simulink model "crc_8_general_manual"  (R2021b)
settings: Solver=FixedStepDiscrete  StartTime=0.0  StopTime=0.01  FixedStep=0.01  RelTol=1e-3
libraries: msbUtilities x9, commcrc2 x1
settings Model: Creator=jekyll  LastModifiedBy=jekyll
settings OptimizationCC: DefaultParameterBehavior=Inlined  EnhancedBackFolding=on  PassReuseOutputArgsAs=Individual arguments  OptimizeBlockOrder=speed  DifferentSizesBufferReuse=on  OptimizationCustomize=off  EfficientTunableParamExpr=on
settings DebuggingCC: ParameterTunabilityLossMsg=error
settings SFSimCC: MATLABDynamicMemAlloc=off
settings RTWCC: Description=Embedded Coder  SystemTargetFile=ert.tlc  GenCodeOnly=on  TemplateMakefile=ert_default_tmf
settings CodeAppCC: ForceParamTrailComments=on  IgnoreCustomStorageClasses=off  OperatorAnnotations=on  SimulinkDataObjDesc=on  SFDataObjDesc=on  InsertBlockDesc=on
settings ERTTargetCC: TargetLangStandard=C99 (ISO)  GenerateSampleERTMain=on  SupportAbsoluteTime=off  CodeInterfacePackaging=Reusable function  SupportNonFinite=off  SupportComplex=off  InlinedParameterPlacement=NonHierarchical  ERTCustomFileTemplate=example_file_process.tlc

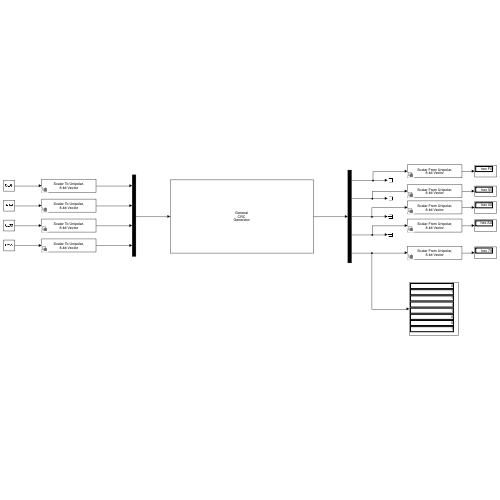
[thumbnail: Simulink's stored preview of the top-level diagram]
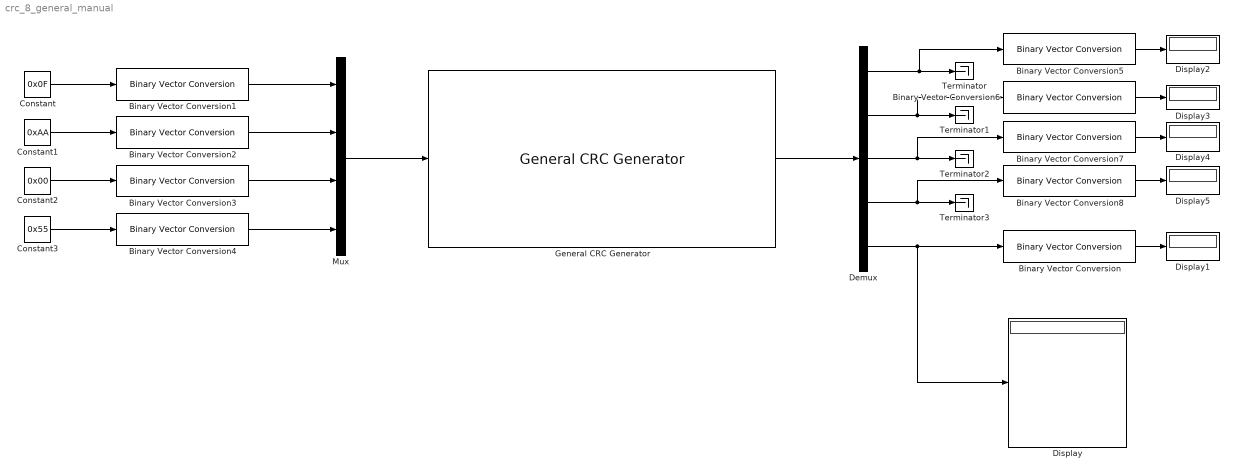
== system crc_8_general_manual ==
  Binary Vector Conversion{,5..8} (5 alike) : msbUtilities/Binary Vector Conversion  LabelModeActiveChoice=From Unipolar  Convert=Binary-coded vector to scalar  Encoding=Unipolar (magnitude)  InputLength=8  InputReverse=MSB at index 1  OutputLength=8  OutputReverse=LSB at index 1  DataType=uint8
      settings: SourceProductBaseCode=AM
  Binary Vector Conversion{1..4} (4 alike) : msbUtilities/Binary Vector Conversion  LabelModeActiveChoice=To Unipolar  Convert=Scalar to binary-coded vector  Encoding=Unipolar (magnitude)  InputLength=8  InputReverse=MSB at index 1  OutputLength=8  OutputReverse=MSB at index 1  DataType=uint8
      settings: SourceProductBaseCode=AM
  Constant : Constant  Value=0x0F  OutDataTypeStr=uint8
  Constant1 : Constant  Value=0xAA  OutDataTypeStr=uint8
  Constant2 : Constant  Value=0x00  OutDataTypeStr=uint8
  Constant3 : Constant  Value=0x55  OutDataTypeStr=uint8
  Demux : Demux  Outputs=5
  Display{,1..5} (6 alike) : Display
      Display settings: Format=decimal (Stored Integer)
      Display1 settings: Format=hex (Stored Integer)
      Display2 settings: Format=hex (Stored Integer)
      Display3 settings: Format=hex (Stored Integer)
      Display4 settings: Format=hex (Stored Integer)
      Display5 settings: Format=hex (Stored Integer)
  General CRC Generator : commcrc2/General CRC Generator  genPoly='z^8 + z^4 + z^3 + z^2 + 1'  iniStates=1  directMethod=on  reflectInputBytes=off  reflectChecksums=off  finalXOR=1  numChecksums=1
      settings: SourceProductBaseCode=CM
  Mux : Mux
  Terminator{,1..3} (4 alike) : Terminator
  wires:
  Demux/5 -> Display/1, Binary Vector Conversion/1
  Demux/3 -> Binary Vector Conversion7/1, Terminator2/1
  Binary Vector Conversion1/1 -> Mux/1
  Binary Vector Conversion4/1 -> Mux/4
  Binary Vector Conversion2/1 -> Mux/2
  Binary Vector Conversion3/1 -> Mux/3
  Demux/2 -> Binary Vector Conversion6/1, Terminator1/1
  Mux/1 -> General CRC Generator/1
  Demux/4 -> Binary Vector Conversion8/1, Terminator3/1
  General CRC Generator/1 -> Demux/1
  Constant/1 -> Binary Vector Conversion1/1
  Constant1/1 -> Binary Vector Conversion2/1
  Constant2/1 -> Binary Vector Conversion3/1
  Constant3/1 -> Binary Vector Conversion4/1
  Demux/1 -> Binary Vector Conversion5/1, Terminator/1
  Binary Vector Conversion/1 -> Display1/1
  Binary Vector Conversion5/1 -> Display2/1
  Binary Vector Conversion6/1 -> Display3/1
  Binary Vector Conversion7/1 -> Display4/1
  Binary Vector Conversion8/1 -> Display5/1
